simulink model "rawmotor_sim"  (Simulink 8.1)
settings: Solver=FixedStepDiscrete  SolverMode=SingleTasking  StartTime=0.0  StopTime=10.0  RelTol=1e-3
libraries: sphero_lib x3
settings Model: Creator=gcampa  LastModifiedBy=gcampa
settings DataIOCC: SignalLoggingSaveFormat=Dataset
settings OptimizationCC: BlockReduction=off  BooleanDataType=off  ExpressionDepthLimit=128
settings DebuggingCC: SaveWithParameterizedLinksMsg=none  SignalResolutionControl=TryResolveAllWithWarning  SolverPrmCheckMsg=none  FcnCallInpInsideContextMsg=EnableAllAsError  StateNameClashWarn=none
settings HardwareCC: TargetUnknown=on
settings GRTTargetCC: CodeReplacementLibrary=C89/C90 (ANSI)  CombineOutputUpdateFcns=on  GRTInterface=off

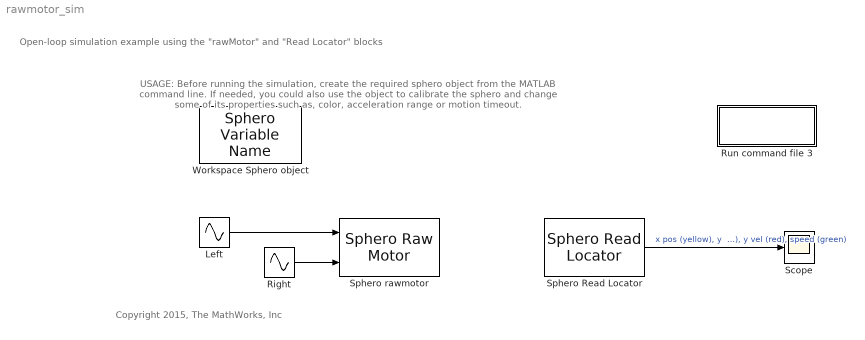
== system rawmotor_sim ==
  note: Copyright 2015, The MathWorks, Inc
  note: USAGE:
      | Before running the simulation, create the required sphero object
      | from the MATLAB command line. If needed, you could also use
      | the object to calibrate the sphero and change some of its properties
      | such as, color, acceleration range or motion timeout.
  note: Open-loop simulation example using the "rawMotor" and "Read Locator" blocks
  Left : Sin  Amplitude=100  Frequency=pi/2/5  SampleTime=1
  Right : Sin  Amplitude=100  Frequency=pi/2/5  Phase=pi/2  SampleTime=1
  Run command file 3 : Subsystem
      settings: OpenFcn=sphero_lib
      mask Display: disp('Open Main\nSimulink Library')
  Scope : Scope
      settings: TimeRange=10  YMin=-400  YMax=400  SaveName=yout
  Sphero Read Locator : sphero_lib/Sphero Read Locator  SpheroVarNumber=Existing workspace Sphero variable #1  T=1
  Sphero rawmotor : sphero_lib/Sphero Raw Motor  SpheroVarNumber=Existing workspace Sphero variable #1  T=1
  Workspace Sphero object : sphero_lib/Sphero Variable Name  Priority=3  SpheroVarNumber=Existing workspace Sphero variable #1  workspaceVarName=sph
  wires:
  Sphero Read Locator/1 -> Scope/1  "x pos (yellow), y  pos (magenta), x vel (cyan), y vel (red), speed (green)"
  Right/1 -> Sphero rawmotor/2
  Left/1 -> Sphero rawmotor/1

== system rawmotor_sim/Run command file 3 ==
